simulink library "halin"  (R2021b)
settings: Solver=VariableStepAuto  StartTime=0.0  StopTime=10.0  RelTol=1e-3
undefined symbols (not defined in the file): TRUE
libraries: FVT_lib x37, hcu_lib x31
(part 1 of 4)
settings Model: Creator=13168  LastModifiedBy=FVT23010
settings SolverCC: AlgebraicLoopSolver=TrustRegion
settings DataIOCC: SaveFormat=Array  SignalLoggingSaveFormat=ModelDataLogs  ReturnWorkspaceOutputs=off
settings OptimizationCC: BlockReduction=off  BooleanDataType=off
settings DebuggingCC: SaveWithParameterizedLinksMsg=none  UnderspecifiedInitializationDetection=Classic  MergeDetectMultiDrivingBlocksExec=none  SignalResolutionControl=TryResolveAllWithWarning  SFMachineParentedDataDiag=warning
settings HardwareCC: TargetUnknown=on
settings ModelReferenceCC: PropagateSignalLabelsOutOfModel=off
settings ConfigComp: CovMetricSettings=dw  CovSaveCumulativeToWorkspaceVar=on  CovSaveSingleToWorkspaceVar=on

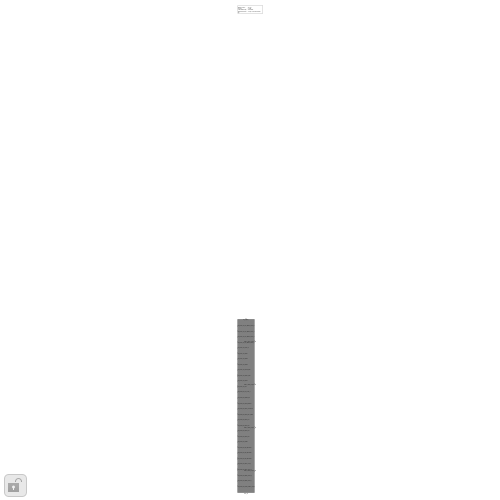
[thumbnail: Simulink's stored preview of the top-level diagram]
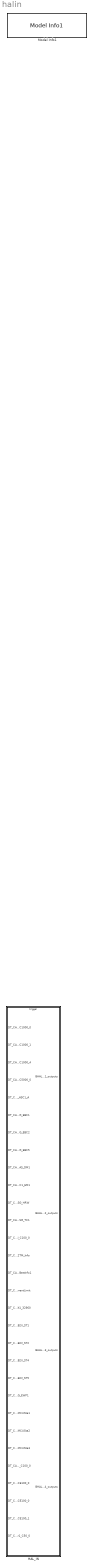
== system halin ==
  HAL_IN : Subsystem
      settings: RTWSystemCode=Nonreusable function  RTWFcnNameOpts=Use subsystem name  RTWFileNameOpts=Use subsystem name
  Model Info1 : hcu_lib/Model Info1  BlockCM=None  Frame=on  DisplayStringWithTags=|  HorizontalTextAlignment=Left  LeftAlignmentValue=0.02  SourceBlockDiagram=hcu_lib  TagMaxNumber=20
      | Model Version        : %<ModelVersion>
      | Creator                   : %<Creator>
      | Last Modified By    : %<LastModifiedBy>
      | Modification date    : %<LastModificationDate>
      settings: SourceProductName=HCU Relative Block Library

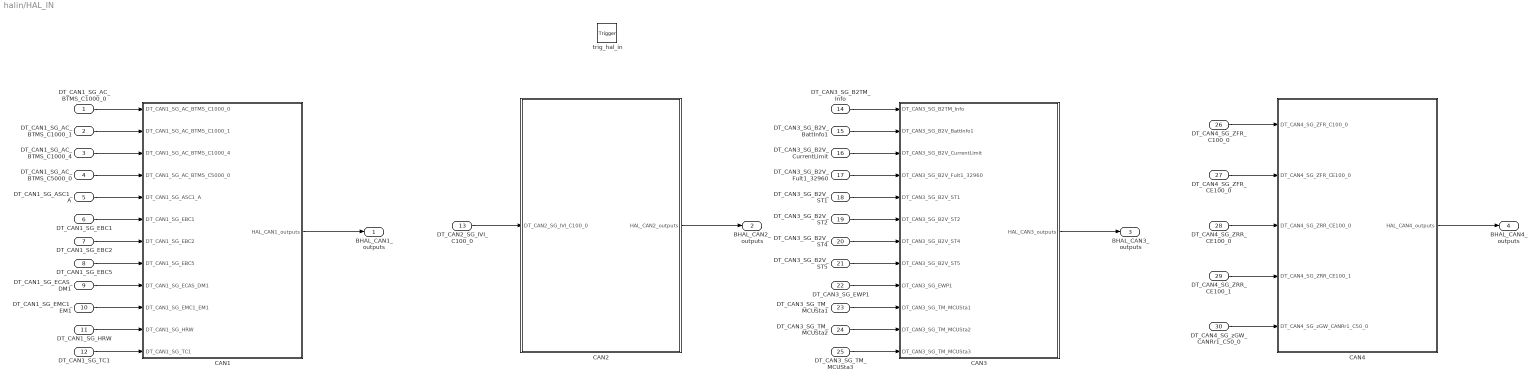
== system halin/HAL_IN ==
  DT_CAN1_SG_AC_BTMS_C1000_0 : Inport
  DT_CAN1_SG_AC_BTMS_C1000_1 : Inport  Port=2
  DT_CAN1_SG_AC_BTMS_C1000_4 : Inport  Port=3
  DT_CAN1_SG_AC_BTMS_C5000_0 : Inport  Port=4
  DT_CAN1_SG_ASC1_A : Inport  Port=5
  DT_CAN1_SG_EBC1 : Inport  Port=6
  DT_CAN1_SG_EBC2 : Inport  Port=7
  DT_CAN1_SG_EBC5 : Inport  Port=8
  DT_CAN1_SG_ECAS_DM1 : Inport  Port=9
  DT_CAN1_SG_EMC1_EM1 : Inport  Port=10
  DT_CAN1_SG_HRW : Inport  Port=11
  DT_CAN1_SG_TC1 : Inport  Port=12
  DT_CAN2_SG_IVI_C100_0 : Inport  Port=13
  DT_CAN3_SG_B2TM_Info : Inport  Port=14
  DT_CAN3_SG_B2V_BattInfo1 : Inport  Port=15
  DT_CAN3_SG_B2V_CurrentLimit : Inport  Port=16
  DT_CAN3_SG_B2V_Fult1_32960 : Inport  Port=17
  DT_CAN3_SG_B2V_ST1 : Inport  Port=18
  DT_CAN3_SG_B2V_ST2 : Inport  Port=19
  DT_CAN3_SG_B2V_ST4 : Inport  Port=20
  DT_CAN3_SG_B2V_ST5 : Inport  Port=21
  DT_CAN3_SG_EWP1 : Inport  Port=22
  DT_CAN3_SG_TM_MCUSta1 : Inport  Port=23
  DT_CAN3_SG_TM_MCUSta2 : Inport  Port=24
  DT_CAN3_SG_TM_MCUSta3 : Inport  Port=25
  DT_CAN4_SG_ZFR_C100_0 : Inport  Port=26
  DT_CAN4_SG_ZFR_CE100_0 : Inport  Port=27
  DT_CAN4_SG_ZRR_CE100_0 : Inport  Port=28
  DT_CAN4_SG_ZRR_CE100_1 : Inport  Port=29
  DT_CAN4_SG_zGW_CANRr1_C50_0 : Inport  Port=30
  trig_hal_in : TriggerPort  TriggerType=function-call  VariantControl=(inherit)
  CAN1 : Subsystem
  CAN2 : Subsystem
  CAN3 : Subsystem
  CAN4 : Subsystem
  BHAL_CAN1_outputs : Outport  OutDataTypeStr=Bus: BHAL_CAN1_outputs
  BHAL_CAN2_outputs : Outport  Port=2  OutDataTypeStr=Bus: BHAL_CAN2_outputs
  BHAL_CAN3_outputs : Outport  Port=3  OutDataTypeStr=Bus: BHAL_CAN3_outputs
  BHAL_CAN4_outputs : Outport  Port=4  OutDataTypeStr=Bus: BHAL_CAN4_outputs
  wires:
  DT_CAN3_SG_TM_MCUSta2/1 -> CAN3/11(DT_CAN3_SG_TM_MCUSta2)
  DT_CAN1_SG_AC_BTMS_C1000_4/1 -> CAN1/3(DT_CAN1_SG_AC_BTMS_C1000_4)
  DT_CAN1_SG_AC_BTMS_C1000_1/1 -> CAN1/2(DT_CAN1_SG_AC_BTMS_C1000_1)
  DT_CAN1_SG_AC_BTMS_C1000_0/1 -> CAN1/1(DT_CAN1_SG_AC_BTMS_C1000_0)
  DT_CAN1_SG_EBC1/1 -> CAN1/6(DT_CAN1_SG_EBC1)
  DT_CAN1_SG_EBC2/1 -> CAN1/7(DT_CAN1_SG_EBC2)
  DT_CAN3_SG_TM_MCUSta3/1 -> CAN3/12(DT_CAN3_SG_TM_MCUSta3)
  DT_CAN1_SG_ASC1_A/1 -> CAN1/5(DT_CAN1_SG_ASC1_A)
  DT_CAN1_SG_HRW/1 -> CAN1/11(DT_CAN1_SG_HRW)
  DT_CAN1_SG_AC_BTMS_C5000_0/1 -> CAN1/4(DT_CAN1_SG_AC_BTMS_C5000_0)
  DT_CAN1_SG_TC1/1 -> CAN1/12(DT_CAN1_SG_TC1)
  DT_CAN1_SG_EMC1_EM1/1 -> CAN1/10(DT_CAN1_SG_EMC1_EM1)
  DT_CAN1_SG_ECAS_DM1/1 -> CAN1/9(DT_CAN1_SG_ECAS_DM1)
  DT_CAN1_SG_EBC5/1 -> CAN1/8(DT_CAN1_SG_EBC5)
  CAN1/1(HAL_CAN1_outputs) -> BHAL_CAN1_outputs/1
  DT_CAN3_SG_B2TM_Info/1 -> CAN3/1(DT_CAN3_SG_B2TM_Info)
  CAN3/1(HAL_CAN3_outputs) -> BHAL_CAN3_outputs/1
  DT_CAN3_SG_B2V_ST5/1 -> CAN3/8(DT_CAN3_SG_B2V_ST5)
  DT_CAN3_SG_B2V_ST4/1 -> CAN3/7(DT_CAN3_SG_B2V_ST4)
  DT_CAN3_SG_B2V_CurrentLimit/1 -> CAN3/3(DT_CAN3_SG_B2V_CurrentLimit)
  DT_CAN3_SG_EWP1/1 -> CAN3/9(DT_CAN3_SG_EWP1)
  CAN2/1(HAL_CAN2_outputs) -> BHAL_CAN2_outputs/1
  DT_CAN3_SG_B2V_ST2/1 -> CAN3/6(DT_CAN3_SG_B2V_ST2)
  DT_CAN3_SG_B2V_ST1/1 -> CAN3/5(DT_CAN3_SG_B2V_ST1)
  DT_CAN4_SG_ZFR_C100_0/1 -> CAN4/1(DT_CAN4_SG_ZFR_C100_0)
  CAN4/1(HAL_CAN4_outputs) -> BHAL_CAN4_outputs/1
  DT_CAN4_SG_ZFR_CE100_0/1 -> CAN4/2(DT_CAN4_SG_ZFR_CE100_0)
  DT_CAN3_SG_TM_MCUSta1/1 -> CAN3/10(DT_CAN3_SG_TM_MCUSta1)
  DT_CAN2_SG_IVI_C100_0/1 -> CAN2/1(DT_CAN2_SG_IVI_C100_0)
  DT_CAN4_SG_zGW_CANRr1_C50_0/1 -> CAN4/5(DT_CAN4_SG_zGW_CANRr1_C50_0)
  DT_CAN4_SG_ZRR_CE100_1/1 -> CAN4/4(DT_CAN4_SG_ZRR_CE100_1)
  DT_CAN4_SG_ZRR_CE100_0/1 -> CAN4/3(DT_CAN4_SG_ZRR_CE100_0)
  DT_CAN3_SG_B2V_Fult1_32960/1 -> CAN3/4(DT_CAN3_SG_B2V_Fult1_32960)
  DT_CAN3_SG_B2V_BattInfo1/1 -> CAN3/2(DT_CAN3_SG_B2V_BattInfo1)

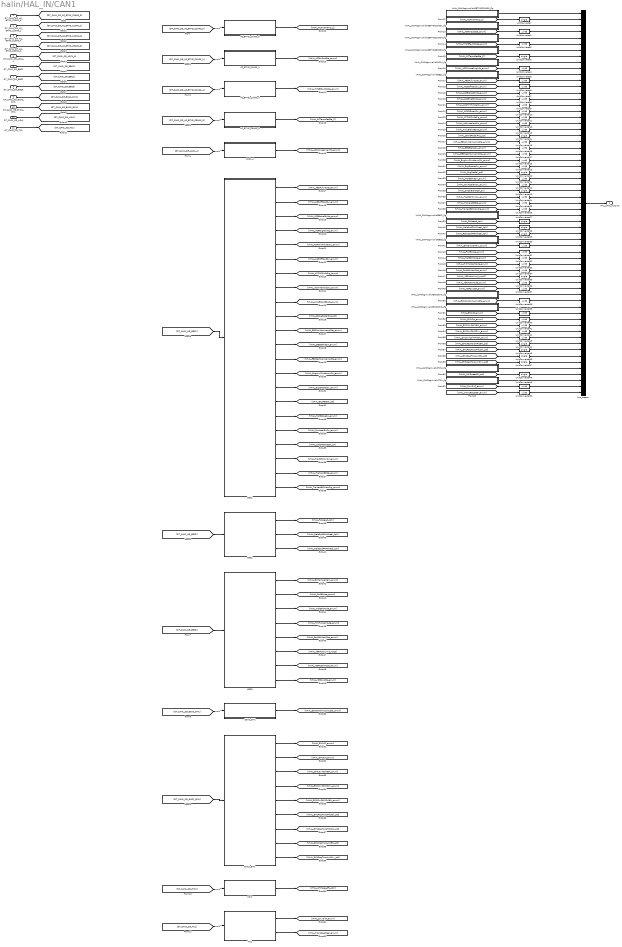
== system halin/HAL_IN/CAN1 ==
  DT_CAN1_SG_AC_BTMS_C1000_0 : Inport
  DT_CAN1_SG_AC_BTMS_C1000_1 : Inport  Port=2
  DT_CAN1_SG_AC_BTMS_C1000_4 : Inport  Port=3
  DT_CAN1_SG_AC_BTMS_C5000_0 : Inport  Port=4
  DT_CAN1_SG_ASC1_A : Inport  Port=5
  DT_CAN1_SG_EBC1 : Inport  Port=6
  DT_CAN1_SG_EBC2 : Inport  Port=7
  DT_CAN1_SG_EBC5 : Inport  Port=8
  DT_CAN1_SG_ECAS_DM1 : Inport  Port=9
  DT_CAN1_SG_EMC1_EM1 : Inport  Port=10
  DT_CAN1_SG_HRW : Inport  Port=11
  DT_CAN1_SG_TC1 : Inport  Port=12
  AC_BTMS_C1000_0 : Subsystem
  AC_BTMS_C1000_1 : Subsystem
  AC_BTMS_C1000_4 : Subsystem
  AC_BTMS_C5000_0 : Subsystem
  ASC1_A : Subsystem
  EBC1 : Subsystem
  EBC2 : Subsystem
  EBC5 : Subsystem
  ECAS_DM1 : Subsystem
  EMC1_EM1 : Subsystem
  HRW : Subsystem
  TC1 : Subsystem
  UnitConverter{,3,14,20,23,27..29,35,44..48} (14 alike) : DataTypeConversion  OutDataTypeStr=single
  UnitConverter{1..2,4..13,15..19,21..22,24..26,30..34,36..43,49..50} (37 alike) : DataTypeConversion  OutDataTypeStr=uint8
  VHAL_CANMsgInvalidACBTMSC10000_flg : Subsystem  AncestorBlock=FVT_lib/hal/MsgTimeoutJudge_CAN_AUTOSAR
      mask help: MeasumentTrigerEvent
      mask Display: fprintf('MsgTimeoutJudge_CAN\nAUTOSAR');
  VHAL_CANMsgInvalidACBTMSC10001_flg : Subsystem  AncestorBlock=FVT_lib/hal/MsgTimeoutJudge_CAN_AUTOSAR
      mask help: MeasumentTrigerEvent
      mask Display: fprintf('MsgTimeoutJudge_CAN\nAUTOSAR');
  VHAL_CANMsgInvalidACBTMSC10004_flg : Subsystem  AncestorBlock=FVT_lib/hal/MsgTimeoutJudge_CAN_AUTOSAR
      mask help: MeasumentTrigerEvent
      mask Display: fprintf('MsgTimeoutJudge_CAN\nAUTOSAR');
  VHAL_CANMsgInvalidACBTMSC50000_flg : Subsystem  AncestorBlock=FVT_lib/hal/MsgTimeoutJudge_CAN_AUTOSAR
      mask help: MeasumentTrigerEvent
      mask Display: fprintf('MsgTimeoutJudge_CAN\nAUTOSAR');
  VHAL_CANMsgInvalidASC1A_flg : Subsystem  AncestorBlock=FVT_lib/hal/MsgTimeoutJudge_CAN_AUTOSAR
      mask help: MeasumentTrigerEvent
      mask Display: fprintf('MsgTimeoutJudge_CAN\nAUTOSAR');
  VHAL_CANMsgInvalidEBC1_flg : Subsystem  AncestorBlock=FVT_lib/hal/MsgTimeoutJudge_CAN_AUTOSAR
      mask help: MeasumentTrigerEvent
      mask Display: fprintf('MsgTimeoutJudge_CAN\nAUTOSAR');
  VHAL_CANMsgInvalidEBC2_flg : Subsystem  AncestorBlock=FVT_lib/hal/MsgTimeoutJudge_CAN_AUTOSAR
      mask help: MeasumentTrigerEvent
      mask Display: fprintf('MsgTimeoutJudge_CAN\nAUTOSAR');
  VHAL_CANMsgInvalidEBC5_flg : Subsystem  AncestorBlock=FVT_lib/hal/MsgTimeoutJudge_CAN_AUTOSAR
      mask help: MeasumentTrigerEvent
      mask Display: fprintf('MsgTimeoutJudge_CAN\nAUTOSAR');
  VHAL_CANMsgInvalidECASDM1_flg : Subsystem  AncestorBlock=FVT_lib/hal/MsgTimeoutJudge_CAN_AUTOSAR
      mask help: MeasumentTrigerEvent
      mask Display: fprintf('MsgTimeoutJudge_CAN\nAUTOSAR');
  VHAL_CANMsgInvalidEMC1EM1_flg : Subsystem  AncestorBlock=FVT_lib/hal/MsgTimeoutJudge_CAN_AUTOSAR
      mask help: MeasumentTrigerEvent
      mask Display: fprintf('MsgTimeoutJudge_CAN\nAUTOSAR');
  VHAL_CANMsgInvalidHRW_flg : Subsystem  AncestorBlock=FVT_lib/hal/MsgTimeoutJudge_CAN_AUTOSAR
      mask help: MeasumentTrigerEvent
      mask Display: fprintf('MsgTimeoutJudge_CAN\nAUTOSAR');
  VHAL_CANMsgInvalidTC1_flg : Subsystem  AncestorBlock=FVT_lib/hal/MsgTimeoutJudge_CAN_AUTOSAR
      mask help: MeasumentTrigerEvent
      mask Display: fprintf('MsgTimeoutJudge_CAN\nAUTOSAR');
  bus_creator : BusCreator  Inputs=63  OutDataTypeStr=Bus: BHAL_CAN1_outputs  NonVirtualBus=on
  HAL_CAN1_outputs : Outport
  wires:
  DT_CAN1_SG_AC_BTMS_C1000_0/1 -> [DT_CAN1_SG_AC_BTMS_C1000_0]
  DT_CAN1_SG_AC_BTMS_C1000_1/1 -> [DT_CAN1_SG_AC_BTMS_C1000_1]
  DT_CAN1_SG_AC_BTMS_C1000_4/1 -> [DT_CAN1_SG_AC_BTMS_C1000_4]
  DT_CAN1_SG_AC_BTMS_C5000_0/1 -> [DT_CAN1_SG_AC_BTMS_C5000_0]
  DT_CAN1_SG_ASC1_A/1 -> [DT_CAN1_SG_ASC1_A]
  DT_CAN1_SG_EBC1/1 -> [DT_CAN1_SG_EBC1]
  DT_CAN1_SG_EBC2/1 -> [DT_CAN1_SG_EBC2]
  DT_CAN1_SG_EBC5/1 -> [DT_CAN1_SG_EBC5]
  DT_CAN1_SG_ECAS_DM1/1 -> [DT_CAN1_SG_ECAS_DM1]
  DT_CAN1_SG_EMC1_EM1/1 -> [DT_CAN1_SG_EMC1_EM1]
  DT_CAN1_SG_HRW/1 -> [DT_CAN1_SG_HRW]
  DT_CAN1_SG_TC1/1 -> [DT_CAN1_SG_TC1]
  [DT_CAN1_SG_AC_BTMS_C1000_0] -> AC_BTMS_C1000_0/1(DT_CAN1_SG_AC_BTMS_C1000_0)
  [DT_CAN1_SG_AC_BTMS_C1000_1] -> AC_BTMS_C1000_1/1(DT_CAN1_SG_AC_BTMS_C1000_1)
  [DT_CAN1_SG_AC_BTMS_C1000_4] -> AC_BTMS_C1000_4/1(DT_CAN1_SG_AC_BTMS_C1000_4)
  [DT_CAN1_SG_AC_BTMS_C5000_0] -> AC_BTMS_C5000_0/1(DT_CAN1_SG_AC_BTMS_C5000_0)
  [DT_CAN1_SG_ASC1_A] -> ASC1_A/1(DT_CAN1_SG_ASC1_A)
  [DT_CAN1_SG_EBC1] -> EBC1/1(DT_CAN1_SG_EBC1)
  [DT_CAN1_SG_EBC2] -> EBC2/1(DT_CAN1_SG_EBC2)
  [DT_CAN1_SG_EBC5] -> EBC5/1(DT_CAN1_SG_EBC5)
  [DT_CAN1_SG_ECAS_DM1] -> ECAS_DM1/1(DT_CAN1_SG_ECAS_DM1)
  [DT_CAN1_SG_EMC1_EM1] -> EMC1_EM1/1(DT_CAN1_SG_EMC1_EM1)
  [DT_CAN1_SG_HRW] -> HRW/1(DT_CAN1_SG_HRW)
  [DT_CAN1_SG_TC1] -> TC1/1(DT_CAN1_SG_TC1)
  bus_creator/1 -> HAL_CAN1_outputs/1
  VHAL_CANMsgInvalidACBTMSC10000_flg/1(Out) -> bus_creator/1
  AC_BTMS_C1000_0/1(VHAL_ACAmbTemp_C) -> [VHAL_ACAmbTemp_C]
  UnitConverter/1 -> bus_creator/2  "VHAL_ACAmbTemp_C"
  [VHAL_ACAmbTemp_C] -> UnitConverter/1
  VHAL_CANMsgInvalidACBTMSC10001_flg/1(Out) -> bus_creator/3
  AC_BTMS_C1000_1/1(VHAL_ACFanSpdSta_enum) -> [VHAL_ACFanSpdSta_enum]
  UnitConverter1/1 -> bus_creator/4  "VHAL_ACFanSpdSta_enum"
  [VHAL_ACFanSpdSta_enum] -> UnitConverter1/1
  VHAL_CANMsgInvalidACBTMSC10004_flg/1(Out) -> bus_creator/5
  AC_BTMS_C1000_4/1(VHAL_TM2BFaultCode_enum) -> [VHAL_TM2BFaultCode_enum]
  UnitConverter2/1 -> bus_creator/6  "VHAL_TM2BFaultCode_enum"
  [VHAL_TM2BFaultCode_enum] -> UnitConverter2/1
  VHAL_CANMsgInvalidACBTMSC50000_flg/1(Out) -> bus_creator/7
  AC_BTMS_C5000_0/1(VHAL_ACTempSetSta_C) -> [VHAL_ACTempSetSta_C]
  UnitConverter3/1 -> bus_creator/8  "VHAL_ACTempSetSta_C"
  [VHAL_ACTempSetSta_C] -> UnitConverter3/1
  VHAL_CANMsgInvalidASC1A_flg/1(Out) -> bus_creator/9
  ASC1_A/1(VHAL_ASC1KneelingInfo_enum) -> [VHAL_ASC1KneelingInfo_enum]
  UnitConverter4/1 -> bus_creator/10  "VHAL_ASC1KneelingInfo_enum"
  [VHAL_ASC1KneelingInfo_enum] -> UnitConverter4/1
  VHAL_CANMsgInvalidEBC1_flg/1(Out) -> bus_creator/11
  EBC1/1(VHAL_ABSFullyOper_enum) -> [VHAL_ABSFullyOper_enum]
  UnitConverter5/1 -> bus_creator/12  "VHAL_ABSFullyOper_enum"
  [VHAL_ABSFullyOper_enum] -> UnitConverter5/1
  EBC1/2(VHAL_ABSOffroadSw_enum) -> [VHAL_ABSOffroadSw_enum]
  UnitConverter6/1 -> bus_creator/13  "VHAL_ABSOffroadSw_enum"
  [VHAL_ABSOffroadSw_enum] -> UnitConverter6/1
  EBC1/3(VHAL_ASRBrakeCtrlAtc_enum) -> [VHAL_ASRBrakeCtrlAtc_enum]
  UnitConverter7/1 -> bus_creator/14  "VHAL_ASRBrakeCtrlAtc_enum"
  [VHAL_ASRBrakeCtrlAtc_enum] -> UnitConverter7/1
  EBC1/4(VHAL_ASREngCtrlAtc_enum) -> [VHAL_ASREngCtrlAtc_enum]
  UnitConverter8/1 -> bus_creator/15  "VHAL_ASREngCtrlAtc_enum"
  [VHAL_ASREngCtrlAtc_enum] -> UnitConverter8/1
  EBC1/5(VHAL_ASRHillHolderSw_enum) -> [VHAL_ASRHillHolderSw_enum]
  UnitConverter9/1 -> bus_creator/16  "VHAL_ASRHillHolderSw_enum"
  [VHAL_ASRHillHolderSw_enum] -> UnitConverter9/1
  EBC1/6(VHAL_ASROffroadSw_enum) -> [VHAL_ASROffroadSw_enum]
  UnitConverter10/1 -> bus_creator/17  "VHAL_ASROffroadSw_enum"
  [VHAL_ASROffroadSw_enum] -> UnitConverter10/1
  EBC1/7(VHAL_ATCASRInfoSig_enum) -> [VHAL_ATCASRInfoSig_enum]
  UnitConverter11/1 -> bus_creator/18  "VHAL_ATCASRInfoSig_enum"
  [VHAL_ATCASRInfoSig_enum] -> UnitConverter11/1
  EBC1/8(VHAL_AcltrInterlockSw_enum) -> [VHAL_AcltrInterlockSw_enum]
  UnitConverter12/1 -> bus_creator/19  "VHAL_AcltrInterlockSw_enum"
  [VHAL_AcltrInterlockSw_enum] -> UnitConverter12/1
  EBC1/9(VHAL_AntiLBrakABSAct_enum) -> [VHAL_AntiLBrakABSAct_enum]
  UnitConverter13/1 -> bus_creator/20  "VHAL_AntiLBrakABSAct_enum"
  [VHAL_AntiLBrakABSAct_enum] -> UnitConverter13/1
  EBC1/10(VHAL_BrakePedalPos_pct) -> [VHAL_BrakePedalPos_pct]
  UnitConverter14/1 -> bus_creator/21  "VHAL_BrakePedalPos_pct"
  [VHAL_BrakePedalPos_pct] -> UnitConverter14/1
  EBC1/11(VHAL_EBSAmWarnLampSta_enum) -> [VHAL_EBSAmWarnLampSta_enum]
  UnitConverter15/1 -> bus_creator/22  "VHAL_EBSAmWarnLampSta_enum"
  [VHAL_EBSAmWarnLampSta_enum] -> UnitConverter15/1
  EBC1/12(VHAL_EBSBrakeSw_enum) -> [VHAL_EBSBrakeSw_enum]
  UnitConverter16/1 -> bus_creator/23  "VHAL_EBSBrakeSw_enum"
  [VHAL_EBSBrakeSw_enum] -> UnitConverter16/1
  EBC1/13(VHAL_EBSRedWarnLampSta_enum) -> [VHAL_EBSRedWarnLampSta_enum]
  UnitConverter17/1 -> bus_creator/24  "VHAL_EBSRedWarnLampSta_enum"
  [VHAL_EBSRedWarnLampSta_enum] -> UnitConverter17/1
  EBC1/14(VHAL_EngAuxShutdownSw_enum) -> [VHAL_EngAuxShutdownSw_enum]
  UnitConverter18/1 -> bus_creator/25  "VHAL_EngAuxShutdownSw_enum"
  [VHAL_EngAuxShutdownSw_enum] -> UnitConverter18/1
  EBC1/15(VHAL_EngDerateSw_enum) -> [VHAL_EngDerateSw_enum]
  UnitConverter19/1 -> bus_creator/26  "VHAL_EngDerateSw_enum"
  [VHAL_EngDerateSw_enum] -> UnitConverter19/1
  EBC1/16(VHAL_EngRetSel_pct) -> [VHAL_EngRetSel_pct]
  UnitConverter20/1 -> bus_creator/27  "VHAL_EngRetSel_pct"
  [VHAL_EngRetSel_pct] -> UnitConverter20/1
  EBC1/17(VHAL_HaltBrakeSw_enum) -> [VHAL_HaltBrakeSw_enum]
  UnitConverter21/1 -> bus_creator/28  "VHAL_HaltBrakeSw_enum"
  [VHAL_HaltBrakeSw_enum] -> UnitConverter21/1
  EBC1/18(VHAL_RmAccelEnSw_enum) -> [VHAL_RmAccelEnSw_enum]
  UnitConverter22/1 -> bus_creator/29  "VHAL_RmAccelEnSw_enum"
  [VHAL_RmAccelEnSw_enum] -> UnitConverter22/1
  EBC1/19(VHAL_SACtrlBrakeCtrl_SA) -> [VHAL_SACtrlBrakeCtrl_SA]
  UnitConverter23/1 -> bus_creator/30  "VHAL_SACtrlBrakeCtrl_SA"
  [VHAL_SACtrlBrakeCtrl_SA] -> UnitConverter23/1
  EBC1/20(VHAL_TractCtrlOvrSw_enum) -> [VHAL_TractCtrlOvrSw_enum]
  UnitConverter24/1 -> bus_creator/31  "VHAL_TractCtrlOvrSw_enum"
  [VHAL_TractCtrlOvrSw_enum] -> UnitConverter24/1
  EBC1/21(VHAL_TrailerABSSta_enum) -> [VHAL_TrailerABSSta_enum]
  UnitConverter25/1 -> bus_creator/32  "VHAL_TrailerABSSta_enum"
  [VHAL_TrailerABSSta_enum] -> UnitConverter25/1
  EBC1/22(VHAL_TrailerABSWarnSig_enum) -> [VHAL_TrailerABSWarnSig_enum]
  UnitConverter26/1 -> bus_creator/33  "VHAL_TrailerABSWarnSig_enum"
  [VHAL_TrailerABSWarnSig_enum] -> UnitConverter26/1
  VHAL_CANMsgInvalidEBC2_flg/1(Out) -> bus_creator/34
  EBC2/1(VHAL_FASpeed_kph) -> [VHAL_FASpeed_kph]
  UnitConverter27/1 -> bus_creator/35  "VHAL_FASpeed_kph"
  [VHAL_FASpeed_kph] -> UnitConverter27/1
  EBC2/2(VHAL_RelaSpdFALWheel_kph) -> [VHAL_RelaSpdFALWheel_kph]
  UnitConverter28/1 -> bus_creator/36  "VHAL_RelaSpdFALWheel_kph"
  [VHAL_RelaSpdFALWheel_kph] -> UnitConverter28/1
  EBC2/3(VHAL_RelaSpdFARWheel_kph) -> [VHAL_RelaSpdFARWheel_kph]
  UnitConverter29/1 -> bus_creator/37  "VHAL_RelaSpdFARWheel_kph"
  [VHAL_RelaSpdFARWheel_kph] -> UnitConverter29/1
  VHAL_CANMsgInvalidEBC5_flg/1(Out) -> bus_creator/38
  EBC5/1(VHAL_BrkTempeWarn_enum) -> [VHAL_BrkTempeWarn_enum]
  UnitConverter30/1 -> bus_creator/39  "VHAL_BrkTempeWarn_enum"
  [VHAL_BrkTempeWarn_enum] -> UnitConverter30/1
  EBC5/2(VHAL_FndBrkUse_enum) -> [VHAL_FndBrkUse_enum]
  UnitConverter31/1 -> bus_creator/40  "VHAL_FndBrkUse_enum"
  [VHAL_FndBrkUse_enum] -> UnitConverter31/1
  EBC5/3(VHAL_HaltBrkMode_enum) -> [VHAL_HaltBrkMode_enum]
  UnitConverter32/1 -> bus_creator/41  "VHAL_HaltBrkMode_enum"
  [VHAL_HaltBrkMode_enum] -> UnitConverter32/1
  EBC5/4(VHAL_HillHolderMode_enum) -> [VHAL_HillHolderMode_enum]
  UnitConverter33/1 -> bus_creator/42  "VHAL_HillHolderMode_enum"
  [VHAL_HillHolderMode_enum] -> UnitConverter33/1
  EBC5/5(VHAL_ParkBrkActuFAct_enum) -> [VHAL_ParkBrkActuFAct_enum]
  UnitConverter34/1 -> bus_creator/43  "VHAL_ParkBrkActuFAct_enum"
  [VHAL_ParkBrkActuFAct_enum] -> UnitConverter34/1
  EBC5/6(VHAL_XBRAcltnLimit_mps2) -> [VHAL_XBRAcltnLimit_mps2]
  UnitConverter35/1 -> bus_creator/44  "VHAL_XBRAcltnLimit_mps2"
  [VHAL_XBRAcltnLimit_mps2] -> UnitConverter35/1
  EBC5/7(VHAL_XBRActtrlMode_enum) -> [VHAL_XBRActtrlMode_enum]
  UnitConverter36/1 -> bus_creator/45  "VHAL_XBRActtrlMode_enum"
  [VHAL_XBRActtrlMode_enum] -> UnitConverter36/1
  EBC5/8(VHAL_XBRSysSta_enum) -> [VHAL_XBRSysSta_enum]
  UnitConverter37/1 -> bus_creator/46  "VHAL_XBRSysSta_enum"
  [VHAL_XBRSysSta_enum] -> UnitConverter37/1
  VHAL_CANMsgInvalidECASDM1_flg/1(Out) -> bus_creator/47
  ECAS_DM1/1(VHAL_ECASAWarmLampSta_enum) -> [VHAL_ECASAWarmLampSta_enum]
  UnitConverter38/1 -> bus_creator/48  "VHAL_ECASAWarmLampSta_enum"
  [VHAL_ECASAWarmLampSta_enum] -> UnitConverter38/1
  VHAL_CANMsgInvalidEMC1EM1_flg/1(Out) -> bus_creator/49
  EMC1_EM1/1(VHAL_EM1CS_enum) -> [VHAL_EM1CS_enum]
  UnitConverter39/1 -> bus_creator/50  "VHAL_EM1CS_enum"
  [VHAL_EM1CS_enum] -> UnitConverter39/1
  EMC1_EM1/2(VHAL_EM1Cnt_enum) -> [VHAL_EM1Cnt_enum]
  UnitConverter40/1 -> bus_creator/51  "VHAL_EM1Cnt_enum"
  [VHAL_EM1Cnt_enum] -> UnitConverter40/1
  EMC1_EM1/3(VHAL_EM1OvrCtrlMBrk_enum) -> [VHAL_EM1OvrCtrlMBrk_enum]
  UnitConverter41/1 -> bus_creator/52  "VHAL_EM1OvrCtrlMBrk_enum"
  [VHAL_EM1OvrCtrlMBrk_enum] -> UnitConverter41/1
  EMC1_EM1/4(VHAL_EM1OvrCtrlMDriv_enum) -> [VHAL_EM1OvrCtrlMDriv_enum]
  UnitConverter42/1 -> bus_creator/53  "VHAL_EM1OvrCtrlMDriv_enum"
  [VHAL_EM1OvrCtrlMDriv_enum] -> UnitConverter42/1
  EMC1_EM1/5(VHAL_EM1OvrCtrlMPriBrk_enum) -> [VHAL_EM1OvrCtrlMPriBrk_enum]
  UnitConverter43/1 -> bus_creator/54  "VHAL_EM1OvrCtrlMPriBrk_enum"
  [VHAL_EM1OvrCtrlMPriBrk_enum] -> UnitConverter43/1
  EMC1_EM1/6(VHAL_EM1ReqTorqHRlsBrk_pct) -> [VHAL_EM1ReqTorqHRlsBrk_pct]
  UnitConverter44/1 -> bus_creator/55  "VHAL_EM1ReqTorqHRlsBrk_pct"
  [VHAL_EM1ReqTorqHRlsBrk_pct] -> UnitConverter44/1
  EMC1_EM1/7(VHAL_EM1ReqTorqHRlsDri_pct) -> [VHAL_EM1ReqTorqHRlsDri_pct]
  UnitConverter45/1 -> bus_creator/56  "VHAL_EM1ReqTorqHRlsDri_pct"
  [VHAL_EM1ReqTorqHRlsDri_pct] -> UnitConverter45/1
  EMC1_EM1/8(VHAL_EM1ReqTorqLimBrk_pct) -> [VHAL_EM1ReqTorqLimBrk_pct]
  UnitConverter46/1 -> bus_creator/57  "VHAL_EM1ReqTorqLimBrk_pct"
  [VHAL_EM1ReqTorqLimBrk_pct] -> UnitConverter46/1
  EMC1_EM1/9(VHAL_EM1ReqTorqLimDriv_pct) -> [VHAL_EM1ReqTorqLimDriv_pct]
  UnitConverter47/1 -> bus_creator/58  "VHAL_EM1ReqTorqLimDriv_pct"
  [VHAL_EM1ReqTorqLimDriv_pct] -> UnitConverter47/1
  VHAL_CANMsgInvalidHRW_flg/1(Out) -> bus_creator/59
  HRW/1(VHAL_WhlSpeedFL_kph) -> [VHAL_WhlSpeedFL_kph]
  UnitConverter48/1 -> bus_creator/60  "VHAL_WhlSpeedFL_kph"
  [VHAL_WhlSpeedFL_kph] -> UnitConverter48/1
  VHAL_CANMsgInvalidTC1_flg/1(Out) -> bus_creator/61
  TC1/1(VHAL_DrivDirF_enum) -> [VHAL_DrivDirF_enum]
  UnitConverter49/1 -> bus_creator/62  "VHAL_DrivDirF_enum"
  [VHAL_DrivDirF_enum] -> UnitConverter49/1
  TC1/2(VHAL_TransReqGear_enum) -> [VHAL_TransReqGear_enum]
  UnitConverter50/1 -> bus_creator/63  "VHAL_TransReqGear_enum"
  [VHAL_TransReqGear_enum] -> UnitConverter50/1

== system halin/HAL_IN/CAN2 ==
  DT_CAN2_SG_IVI_C100_0 : Inport
  IVI_C100_0 : Subsystem
  UnitConverter : DataTypeConversion  OutDataTypeStr=uint8
  VHAL_CANMsgInvalidIVIC1000_flg : Subsystem  AncestorBlock=FVT_lib/hal/MsgTimeoutJudge_CAN_AUTOSAR
      mask help: MeasumentTrigerEvent
      mask Display: fprintf('MsgTimeoutJudge_CAN\nAUTOSAR');
  bus_creator : BusCreator  Inputs=2  OutDataTypeStr=Bus: BHAL_CAN2_outputs  NonVirtualBus=on
  HAL_CAN2_outputs : Outport
  wires:
  DT_CAN2_SG_IVI_C100_0/1 -> [DT_CAN2_SG_IVI_C100_0]
  [DT_CAN2_SG_IVI_C100_0] -> IVI_C100_0/1(DT_CAN2_SG_IVI_C100_0)
  bus_creator/1 -> HAL_CAN2_outputs/1
  VHAL_CANMsgInvalidIVIC1000_flg/1(Out) -> bus_creator/1
  IVI_C100_0/1(VHAL_IVIACFanSpdReqCmd_enum) -> [VHAL_IVIACFanSpdReqCmd_enum]
  UnitConverter/1 -> bus_creator/2  "VHAL_IVIACFanSpdReqCmd_enum"
  [VHAL_IVIACFanSpdReqCmd_enum] -> UnitConverter/1

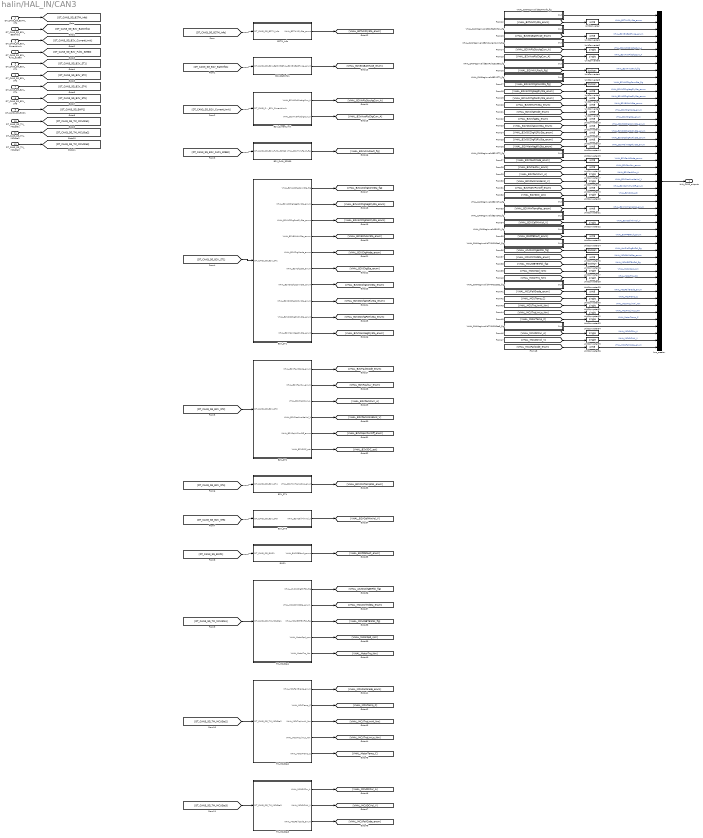
== system halin/HAL_IN/CAN3 ==
  DT_CAN3_SG_B2TM_Info : Inport
  DT_CAN3_SG_B2V_BattInfo1 : Inport  Port=2
  DT_CAN3_SG_B2V_CurrentLimit : Inport  Port=3
  DT_CAN3_SG_B2V_Fult1_32960 : Inport  Port=4
  DT_CAN3_SG_B2V_ST1 : Inport  Port=5
  DT_CAN3_SG_B2V_ST2 : Inport  Port=6
  DT_CAN3_SG_B2V_ST4 : Inport  Port=7
  DT_CAN3_SG_B2V_ST5 : Inport  Port=8
  DT_CAN3_SG_EWP1 : Inport  Port=9
  DT_CAN3_SG_TM_MCUSta1 : Inport  Port=10
  DT_CAN3_SG_TM_MCUSta2 : Inport  Port=11
  DT_CAN3_SG_TM_MCUSta3 : Inport  Port=12
  B2TM_Info : Subsystem
  B2V_BattInfo1 : Subsystem
  B2V_CurrentLimit : Subsystem
  B2V_Fult1_32960 : Subsystem
  B2V_ST1 : Subsystem
  B2V_ST2 : Subsystem
  B2V_ST4 : Subsystem
  B2V_ST5 : Subsystem
  EWP1 : Subsystem
  TM_MCUSta1 : Subsystem
  TM_MCUSta2 : Subsystem
  TM_MCUSta3 : Subsystem
  UnitConverter{,1,6..16,19,21,23,25,29,36} (19 alike) : DataTypeConversion  OutDataTypeStr=uint8
  UnitConverter{2..3,17..18,20,22,27..28,30..35} (14 alike) : DataTypeConversion  OutDataTypeStr=single
  UnitConverter{4..5,24,26} (4 alike) : DataTypeConversion  OutDataTypeStr=boolean
  VHAL_CANMsgInvalidB2TMInfo_flg : Subsystem  AncestorBlock=FVT_lib/hal/MsgTimeoutJudge_CAN_AUTOSAR
      mask help: MeasumentTrigerEvent
      mask Display: fprintf('MsgTimeoutJudge_CAN\nAUTOSAR');
  VHAL_CANMsgInvalidB2VBattInfo1_flg : Subsystem  AncestorBlock=FVT_lib/hal/MsgTimeoutJudge_CAN_AUTOSAR
      mask help: MeasumentTrigerEvent
      mask Display: fprintf('MsgTimeoutJudge_CAN\nAUTOSAR');
  VHAL_CANMsgInvalidB2VCurrentLimit_flg : Subsystem  AncestorBlock=FVT_lib/hal/MsgTimeoutJudge_CAN_AUTOSAR
      mask help: MeasumentTrigerEvent
      mask Display: fprintf('MsgTimeoutJudge_CAN\nAUTOSAR');
  VHAL_CANMsgInvalidB2VFult132960_flg : Subsystem  AncestorBlock=FVT_lib/hal/MsgTimeoutJudge_CAN_AUTOSAR
      mask help: MeasumentTrigerEvent
      mask Display: fprintf('MsgTimeoutJudge_CAN\nAUTOSAR');
  VHAL_CANMsgInvalidB2VST1_flg : Subsystem  AncestorBlock=FVT_lib/hal/MsgTimeoutJudge_CAN_AUTOSAR
      mask help: MeasumentTrigerEvent
      mask Display: fprintf('MsgTimeoutJudge_CAN\nAUTOSAR');
  VHAL_CANMsgInvalidB2VST2_flg : Subsystem  AncestorBlock=FVT_lib/hal/MsgTimeoutJudge_CAN_AUTOSAR
      mask help: MeasumentTrigerEvent
      mask Display: fprintf('MsgTimeoutJudge_CAN\nAUTOSAR');
  VHAL_CANMsgInvalidB2VST4_flg : Subsystem  AncestorBlock=FVT_lib/hal/MsgTimeoutJudge_CAN_AUTOSAR
      mask help: MeasumentTrigerEvent
      mask Display: fprintf('MsgTimeoutJudge_CAN\nAUTOSAR');
  VHAL_CANMsgInvalidB2VST5_flg : Subsystem  AncestorBlock=FVT_lib/hal/MsgTimeoutJudge_CAN_AUTOSAR
      mask help: MeasumentTrigerEvent
      mask Display: fprintf('MsgTimeoutJudge_CAN\nAUTOSAR');
  VHAL_CANMsgInvalidEWP1_flg : Subsystem  AncestorBlock=FVT_lib/hal/MsgTimeoutJudge_CAN_AUTOSAR
      mask help: MeasumentTrigerEvent
      mask Display: fprintf('MsgTimeoutJudge_CAN\nAUTOSAR');
  VHAL_CANMsgInvalidTMMCUSta1_flg : Subsystem  AncestorBlock=FVT_lib/hal/MsgTimeoutJudge_CAN_AUTOSAR
      mask help: MeasumentTrigerEvent
      mask Display: fprintf('MsgTimeoutJudge_CAN\nAUTOSAR');
  VHAL_CANMsgInvalidTMMCUSta2_flg : Subsystem  AncestorBlock=FVT_lib/hal/MsgTimeoutJudge_CAN_AUTOSAR
      mask help: MeasumentTrigerEvent
      mask Display: fprintf('MsgTimeoutJudge_CAN\nAUTOSAR');
  VHAL_CANMsgInvalidTMMCUSta3_flg : Subsystem  AncestorBlock=FVT_lib/hal/MsgTimeoutJudge_CAN_AUTOSAR
      mask help: MeasumentTrigerEvent
      mask Display: fprintf('MsgTimeoutJudge_CAN\nAUTOSAR');
  bus_creator : BusCreator  Inputs=49  OutDataTypeStr=Bus: BHAL_CAN3_outputs  NonVirtualBus=on
  HAL_CAN3_outputs : Outport
  wires:
  DT_CAN3_SG_B2TM_Info/1 -> [DT_CAN3_SG_B2TM_Info]
  DT_CAN3_SG_B2V_BattInfo1/1 -> [DT_CAN3_SG_B2V_BattInfo1]
  DT_CAN3_SG_B2V_CurrentLimit/1 -> [DT_CAN3_SG_B2V_CurrentLimit]
  DT_CAN3_SG_B2V_Fult1_32960/1 -> [DT_CAN3_SG_B2V_Fult1_32960]
  DT_CAN3_SG_B2V_ST1/1 -> [DT_CAN3_SG_B2V_ST1]
  DT_CAN3_SG_B2V_ST2/1 -> [DT_CAN3_SG_B2V_ST2]
  DT_CAN3_SG_B2V_ST4/1 -> [DT_CAN3_SG_B2V_ST4]
  DT_CAN3_SG_B2V_ST5/1 -> [DT_CAN3_SG_B2V_ST5]
  DT_CAN3_SG_EWP1/1 -> [DT_CAN3_SG_EWP1]
  DT_CAN3_SG_TM_MCUSta1/1 -> [DT_CAN3_SG_TM_MCUSta1]
  DT_CAN3_SG_TM_MCUSta2/1 -> [DT_CAN3_SG_TM_MCUSta2]
  DT_CAN3_SG_TM_MCUSta3/1 -> [DT_CAN3_SG_TM_MCUSta3]
  [DT_CAN3_SG_B2TM_Info] -> B2TM_Info/1(DT_CAN3_SG_B2TM_Info)
  [DT_CAN3_SG_B2V_BattInfo1] -> B2V_BattInfo1/1(DT_CAN3_SG_B2V_BattInfo1)
  [DT_CAN3_SG_B2V_CurrentLimit] -> B2V_CurrentLimit/1(DT_CAN3_SG_B2V_CurrentLimit)
  [DT_CAN3_SG_B2V_Fult1_32960] -> B2V_Fult1_32960/1(DT_CAN3_SG_B2V_Fult1_32960)
  [DT_CAN3_SG_B2V_ST1] -> B2V_ST1/1(DT_CAN3_SG_B2V_ST1)
  [DT_CAN3_SG_B2V_ST2] -> B2V_ST2/1(DT_CAN3_SG_B2V_ST2)
  [DT_CAN3_SG_B2V_ST4] -> B2V_ST4/1(DT_CAN3_SG_B2V_ST4)
  [DT_CAN3_SG_B2V_ST5] -> B2V_ST5/1(DT_CAN3_SG_B2V_ST5)
  [DT_CAN3_SG_EWP1] -> EWP1/1(DT_CAN3_SG_EWP1)
  [DT_CAN3_SG_TM_MCUSta1] -> TM_MCUSta1/1(DT_CAN3_SG_TM_MCUSta1)
  [DT_CAN3_SG_TM_MCUSta2] -> TM_MCUSta2/1(DT_CAN3_SG_TM_MCUSta2)
  [DT_CAN3_SG_TM_MCUSta3] -> TM_MCUSta3/1(DT_CAN3_SG_TM_MCUSta3)
  bus_creator/1 -> HAL_CAN3_outputs/1
  VHAL_CANMsgInvalidB2TMInfo_flg/1(Out) -> bus_creator/1
  B2TM_Info/1(VHAL_B2THVRlySta_enum) -> [VHAL_B2THVRlySta_enum]
  UnitConverter/1 -> bus_creator/2  "VHAL_B2THVRlySta_enum"
  [VHAL_B2THVRlySta_enum] -> UnitConverter/1
  VHAL_CANMsgInvalidB2VBattInfo1_flg/1(Out) -> bus_creator/3
  B2V_BattInfo1/1(VHAL_B2VBI1BattType_enum) -> [VHAL_B2VBI1BattType_enum]
  UnitConverter1/1 -> bus_creator/4  "VHAL_B2VBI1BattType_enum"
  [VHAL_B2VBI1BattType_enum] -> UnitConverter1/1
  VHAL_CANMsgInvalidB2VCurrentLimit_flg/1(Out) -> bus_creator/5
  B2V_CurrentLimit/1(VHAL_B2VAPlsDischgCurr_A) -> [VHAL_B2VAPlsDischgCurr_A]
  UnitConverter2/1 -> bus_creator/6  "VHAL_B2VAPlsDischgCurr_A"
  [VHAL_B2VAPlsDischgCurr_A] -> UnitConverter2/1
  B2V_CurrentLimit/2(VHAL_B2VAvaPlsChgCurr_A) -> [VHAL_B2VAvaPlsChgCurr_A]
  UnitConverter3/1 -> bus_creator/7  "VHAL_B2VAvaPlsChgCurr_A"
  [VHAL_B2VAvaPlsChgCurr_A] -> UnitConverter3/1
  VHAL_CANMsgInvalidB2VFult132960_flg/1(Out) -> bus_creator/8
  B2V_Fult1_32960/1(VHAL_B2VHVILFault_flg) -> [VHAL_B2VHVILFault_flg]
  UnitConverter4/1 -> bus_creator/9  "VHAL_B2VHVILFault_flg"
  [VHAL_B2VHVILFault_flg] -> UnitConverter4/1
  VHAL_CANMsgInvalidB2VST1_flg/1(Out) -> bus_creator/10
  B2V_ST1/1(VHAL_B2VACChgConnSta_flg) -> [VHAL_B2VACChgConnSta_flg]
  UnitConverter5/1 -> bus_creator/11  "VHAL_B2VACChgConnSta_flg"
  [VHAL_B2VACChgConnSta_flg] -> UnitConverter5/1
  B2V_ST1/2(VHAL_B2VACChgNegRlySta_enum) -> [VHAL_B2VACChgNegRlySta_enum]
  UnitConverter6/1 -> bus_creator/12  "VHAL_B2VACChgNegRlySta_enum"
  [VHAL_B2VACChgNegRlySta_enum] -> UnitConverter6/1
  B2V_ST1/3(VHAL_B2VACChgPosRlySta_enum) -> [VHAL_B2VACChgPosRlySta_enum]
  UnitConverter7/1 -> bus_creator/13  "VHAL_B2VACChgPosRlySta_enum"
  [VHAL_B2VACChgPosRlySta_enum] -> UnitConverter7/1
  B2V_ST1/4(VHAL_B2VBMUHVSta_enum) -> [VHAL_B2VBMUHVSta_enum]
  UnitConverter8/1 -> bus_creator/14  "VHAL_B2VBMUHVSta_enum"
  [VHAL_B2VBMUHVSta_enum] -> UnitConverter8/1
  B2V_ST1/5(VHAL_B2VChgMode_enum) -> [VHAL_B2VChgMode_enum]
  UnitConverter9/1 -> bus_creator/15  "VHAL_B2VChgMode_enum"
  [VHAL_B2VChgMode_enum] -> UnitConverter9/1
  B2V_ST1/6(VHAL_B2VChgSta_enum) -> [VHAL_B2VChgSta_enum]
  UnitConverter10/1 -> bus_creator/16  "VHAL_B2VChgSta_enum"
  [VHAL_B2VChgSta_enum] -> UnitConverter10/1
  B2V_ST1/7(VHAL_B2VDCChgConnSta_enum) -> [VHAL_B2VDCChgConnSta_enum]
  UnitConverter11/1 -> bus_creator/17  "VHAL_B2VDCChgConnSta_enum"
  [VHAL_B2VDCChgConnSta_enum] -> UnitConverter11/1
  B2V_ST1/8(VHAL_B2VDCChgN1RlySta_enum) -> [VHAL_B2VDCChgN1RlySta_enum]
  UnitConverter12/1 -> bus_creator/18  "VHAL_B2VDCChgN1RlySta_enum"
  [VHAL_B2VDCChgN1RlySta_enum] -> UnitConverter12/1
  B2V_ST1/9(VHAL_B2VDCChgP1RlySta_enum) -> [VHAL_B2VDCChgP1RlySta_enum]
  UnitConverter13/1 -> bus_creator/19  "VHAL_B2VDCChgP1RlySta_enum"
  [VHAL_B2VDCChgP1RlySta_enum] -> UnitConverter13/1
  B2V_ST1/10(VHAL_B2VMainNegRlySta_enum) -> [VHAL_B2VMainNegRlySta_enum]
  UnitConverter14/1 -> bus_creator/20  "VHAL_B2VMainNegRlySta_enum"
  [VHAL_B2VMainNegRlySta_enum] -> UnitConverter14/1
  VHAL_CANMsgInvalidB2VST2_flg/1(Out) -> bus_creator/21
  B2V_ST2/1(VHAL_B2VFaultCode_enum) -> [VHAL_B2VFaultCode_enum]
  UnitConverter15/1 -> bus_creator/22  "VHAL_B2VFaultCode_enum"
  [VHAL_B2VFaultCode_enum] -> UnitConverter15/1
  B2V_ST2/2(VHAL_B2VFaultLv_enum) -> [VHAL_B2VFaultLv_enum]
  UnitConverter16/1 -> bus_creator/23  "VHAL_B2VFaultLv_enum"
  [VHAL_B2VFaultLv_enum] -> UnitConverter16/1
  B2V_ST2/3(VHAL_B2VPackCurr_A) -> [VHAL_B2VPackCurr_A]
  UnitConverter17/1 -> bus_creator/24  "VHAL_B2VPackCurr_A"
  [VHAL_B2VPackCurr_A] -> UnitConverter17/1
  B2V_ST2/4(VHAL_B2VPackInsideVol_V) -> [VHAL_B2VPackInsideVol_V]
  UnitConverter18/1 -> bus_creator/25  "VHAL_B2VPackInsideVol_V"
  [VHAL_B2VPackInsideVol_V] -> UnitConverter18/1
  B2V_ST2/5(VHAL_B2VRqHVPwrOff_enum) -> [VHAL_B2VRqHVPwrOff_enum]
  UnitConverter19/1 -> bus_creator/26  "VHAL_B2VRqHVPwrOff_enum"
  [VHAL_B2VRqHVPwrOff_enum] -> UnitConverter19/1
  B2V_ST2/6(VHAL_B2VSOC_pct) -> [VHAL_B2VSOC_pct]
  UnitConverter20/1 -> bus_creator/27  "VHAL_B2VSOC_pct"
  [VHAL_B2VSOC_pct] -> UnitConverter20/1
  VHAL_CANMsgInvalidB2VST4_flg/1(Out) -> bus_creator/28
  B2V_ST4/1(VHAL_B2VMinTempPos_enum) -> [VHAL_B2VMinTempPos_enum]
  UnitConverter21/1 -> bus_creator/29  "VHAL_B2VMinTempPos_enum"
  [VHAL_B2VMinTempPos_enum] -> UnitConverter21/1
  VHAL_CANMsgInvalidB2VST5_flg/1(Out) -> bus_creator/30
  B2V_ST5/1(VHAL_B2VCellMinVol_V) -> [VHAL_B2VCellMinVol_V]
  UnitConverter22/1 -> bus_creator/31  "VHAL_B2VCellMinVol_V"
  [VHAL_B2VCellMinVol_V] -> UnitConverter22/1
  VHAL_CANMsgInvalidEWP1_flg/1(Out) -> bus_creator/32
  EWP1/1(VHAL_EWPPEFault_enum) -> [VHAL_EWPPEFault_enum]
  UnitConverter23/1 -> bus_creator/33  "VHAL_EWPPEFault_enum"
  [VHAL_EWPPEFault_enum] -> UnitConverter23/1
  VHAL_CANMsgInvalidTMMCUSta1_flg/1(Out) -> bus_creator/34
  TM_MCUSta1/1(VHAL_AtvDisChgEnFbk_flg) -> [VHAL_AtvDisChgEnFbk_flg]
  UnitConverter24/1 -> bus_creator/35  "VHAL_AtvDisChgEnFbk_flg"
  [VHAL_AtvDisChgEnFbk_flg] -> UnitConverter24/1
  TM_MCUSta1/2(VHAL_MCUCtrlMdSta_enum) -> [VHAL_MCUCtrlMdSta_enum]
  UnitConverter25/1 -> bus_creator/36  "VHAL_MCUCtrlMdSta_enum"
  [VHAL_MCUCtrlMdSta_enum] -> UnitConverter25/1
  TM_MCUSta1/3(VHAL_MCUIGBTEnFbk_flg) -> [VHAL_MCUIGBTEnFbk_flg]
  UnitConverter26/1 -> bus_creator/37  "VHAL_MCUIGBTEnFbk_flg"
  [VHAL_MCUIGBTEnFbk_flg] -> UnitConverter26/1
  TM_MCUSta1/4(VHAL_MotorSpd_rpm) -> [VHAL_MotorSpd_rpm]
  UnitConverter27/1 -> bus_creator/38  "VHAL_MotorSpd_rpm"
  [VHAL_MotorSpd_rpm] -> UnitConverter27/1
  TM_MCUSta1/5(VHAL_MotorTrq_Nm) -> [VHAL_MotorTrq_Nm]
  UnitConverter28/1 -> bus_creator/39  "VHAL_MotorTrq_Nm"
  [VHAL_MotorTrq_Nm] -> UnitConverter28/1
  VHAL_CANMsgInvalidTMMCUSta2_flg/1(Out) -> bus_creator/40
  TM_MCUSta2/1(VHAL_MCUFailGrade_enum) -> [VHAL_MCUFailGrade_enum]
  UnitConverter29/1 -> bus_creator/41  "VHAL_MCUFailGrade_enum"
  [VHAL_MCUFailGrade_enum] -> UnitConverter29/1
  TM_MCUSta2/2(VHAL_MCUTemp_C) -> [VHAL_MCUTemp_C]
  UnitConverter30/1 -> bus_creator/42  "VHAL_MCUTemp_C"
  [VHAL_MCUTemp_C] -> UnitConverter30/1
  TM_MCUSta2/3(VHAL_MCUTrqLimHi_Nm) -> [VHAL_MCUTrqLimHi_Nm]
  UnitConverter31/1 -> bus_creator/43  "VHAL_MCUTrqLimHi_Nm"
  [VHAL_MCUTrqLimHi_Nm] -> UnitConverter31/1
  TM_MCUSta2/4(VHAL_MCUTrqLimLo_Nm) -> [VHAL_MCUTrqLimLo_Nm]
  UnitConverter32/1 -> bus_creator/44  "VHAL_MCUTrqLimLo_Nm"
  [VHAL_MCUTrqLimLo_Nm] -> UnitConverter32/1
  TM_MCUSta2/5(VHAL_MotorTemp_C) -> [VHAL_MotorTemp_C]
  UnitConverter33/1 -> bus_creator/45  "VHAL_MotorTemp_C"
  [VHAL_MotorTemp_C] -> UnitConverter33/1
  VHAL_CANMsgInvalidTMMCUSta3_flg/1(Out) -> bus_creator/46
  TM_MCUSta3/1(VHAL_MCUDCCur_A) -> [VHAL_MCUDCCur_A]
  UnitConverter34/1 -> bus_creator/47  "VHAL_MCUDCCur_A"
  [VHAL_MCUDCCur_A] -> UnitConverter34/1
  TM_MCUSta3/2(VHAL_MCUDCVol_V) -> [VHAL_MCUDCVol_V]
  UnitConverter35/1 -> bus_creator/48  "VHAL_MCUDCVol_V"
  [VHAL_MCUDCVol_V] -> UnitConverter35/1
  TM_MCUSta3/3(VHAL_MCUFailCode_enum) -> [VHAL_MCUFailCode_enum]
  UnitConverter36/1 -> bus_creator/49  "VHAL_MCUFailCode_enum"
  [VHAL_MCUFailCode_enum] -> UnitConverter36/1

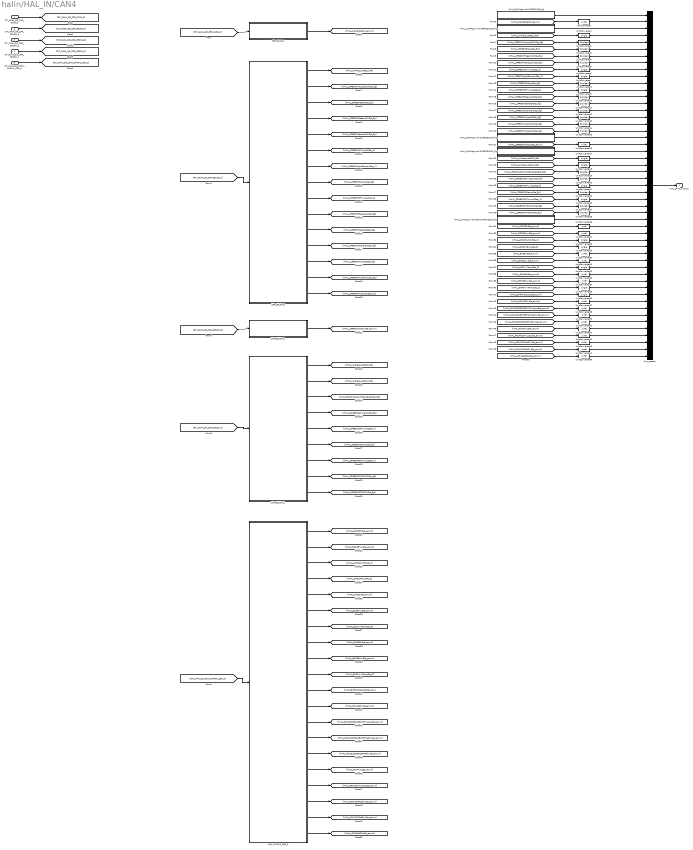
== system halin/HAL_IN/CAN4 ==
  DT_CAN4_SG_ZFR_C100_0 : Inport
  DT_CAN4_SG_ZFR_CE100_0 : Inport  Port=2
  DT_CAN4_SG_ZRR_CE100_0 : Inport  Port=3
  DT_CAN4_SG_ZRR_CE100_1 : Inport  Port=4
  DT_CAN4_SG_zGW_CANRr1_C50_0 : Inport  Port=5
  UnitConverter{,16,26..27,30..31,33..34,37..45} (17 alike) : DataTypeConversion  OutDataTypeStr=uint8
  UnitConverter{1,6..7,9,17..18,21,23,28..29,32,35..36} (13 alike) : DataTypeConversion  OutDataTypeStr=single
  UnitConverter{2..5,8,10..15,19..20,22,24..25} (16 alike) : DataTypeConversion  OutDataTypeStr=boolean
  VHAL_CANMsgInvalidZFRC1000_flg : Subsystem  AncestorBlock=FVT_lib/hal/MsgTimeoutJudge_CAN_AUTOSAR
      mask help: MeasumentTrigerEvent
      mask Display: fprintf('MsgTimeoutJudge_CAN\nAUTOSAR');
  VHAL_CANMsgInvalidZFRCE1000_flg : Subsystem  AncestorBlock=FVT_lib/hal/MsgTimeoutJudge_CAN_AUTOSAR
      mask help: MeasumentTrigerEvent
      mask Display: fprintf('MsgTimeoutJudge_CAN\nAUTOSAR');
  VHAL_CANMsgInvalidZRRCE1000_flg : Subsystem  AncestorBlock=FVT_lib/hal/MsgTimeoutJudge_CAN_AUTOSAR
      mask help: MeasumentTrigerEvent
      mask Display: fprintf('MsgTimeoutJudge_CAN\nAUTOSAR');
  VHAL_CANMsgInvalidZRRCE1001_flg : Subsystem  AncestorBlock=FVT_lib/hal/MsgTimeoutJudge_CAN_AUTOSAR
      mask help: MeasumentTrigerEvent
      mask Display: fprintf('MsgTimeoutJudge_CAN\nAUTOSAR');
  VHAL_CANMsgInvalidzGWCANRr1C500_flg : Subsystem  AncestorBlock=FVT_lib/hal/MsgTimeoutJudge_CAN_AUTOSAR
      mask help: MeasumentTrigerEvent
      mask Display: fprintf('MsgTimeoutJudge_CAN\nAUTOSAR');
  ZFR_C100_0 : Subsystem
  ZFR_CE100_0 : Subsystem
  ZRR_CE100_0 : Subsystem
  ZRR_CE100_1 : Subsystem
  bus_creator : BusCreator  Inputs=51  OutDataTypeStr=Bus: BHAL_CAN4_outputs  NonVirtualBus=on
  zGW_CANRr1_C50_0 : Subsystem
  HAL_CAN4_outputs : Outport
  wires:
  DT_CAN4_SG_ZFR_C100_0/1 -> [DT_CAN4_SG_ZFR_C100_0]
  DT_CAN4_SG_ZFR_CE100_0/1 -> [DT_CAN4_SG_ZFR_CE100_0]
  DT_CAN4_SG_ZRR_CE100_0/1 -> [DT_CAN4_SG_ZRR_CE100_0]
  DT_CAN4_SG_ZRR_CE100_1/1 -> [DT_CAN4_SG_ZRR_CE100_1]
  DT_CAN4_SG_zGW_CANRr1_C50_0/1 -> [DT_CAN4_SG_zGW_CANRr1_C50_0]
  [DT_CAN4_SG_ZFR_C100_0] -> ZFR_C100_0/1(DT_CAN4_SG_ZFR_C100_0)
  [DT_CAN4_SG_ZFR_CE100_0] -> ZFR_CE100_0/1(DT_CAN4_SG_ZFR_CE100_0)
  [DT_CAN4_SG_ZRR_CE100_0] -> ZRR_CE100_0/1(DT_CAN4_SG_ZRR_CE100_0)
  [DT_CAN4_SG_ZRR_CE100_1] -> ZRR_CE100_1/1(DT_CAN4_SG_ZRR_CE100_1)
  [DT_CAN4_SG_zGW_CANRr1_C50_0] -> zGW_CANRr1_C50_0/1(DT_CAN4_SG_zGW_CANRr1_C50_0)
  bus_creator/1 -> HAL_CAN4_outputs/1
  VHAL_CANMsgInvalidZFRC1000_flg/1(Out) -> bus_creator/1
  ZFR_C100_0/1(VHAL_ParkBrakeSW_enum) -> [VHAL_ParkBrakeSW_enum]
  UnitConverter/1 -> bus_creator/2  "VHAL_ParkBrakeSW_enum"
  [VHAL_ParkBrakeSW_enum] -> UnitConverter/1
  VHAL_CANMsgInvalidZFRCE1000_flg/1(Out) -> bus_creator/3
  ZFR_CE100_0/1(VHAL_AirPressureFC2_kPa) -> [VHAL_AirPressureFC2_kPa]
  UnitConverter1/1 -> bus_creator/4  "VHAL_AirPressureFC2_kPa"
  [VHAL_AirPressureFC2_kPa] -> UnitConverter1/1
  ZFR_CE100_0/2(VHAL_ZFRBCMAutoLightSWSta_flg) -> [VHAL_ZFRBCMAutoLightSWSta_flg]
  UnitConverter2/1 -> bus_creator/5  "VHAL_ZFRBCMAutoLightSWSta_flg"
  [VHAL_ZFRBCMAutoLightSWSta_flg] -> UnitConverter2/1
  ZFR_CE100_0/3(VHAL_ZFRBCMBrakeSta_flg) -> [VHAL_ZFRBCMBrakeSta_flg]
  UnitConverter3/1 -> bus_creator/6  "VHAL_ZFRBCMBrakeSta_flg"
  [VHAL_ZFRBCMBrakeSta_flg] -> UnitConverter3/1
  ZFR_CE100_0/4(VHAL_ZFRBCMHBeamSWSta_flg) -> [VHAL_ZFRBCMHBeamSWSta_flg]
  UnitConverter4/1 -> bus_creator/7  "VHAL_ZFRBCMHBeamSWSta_flg"
  [VHAL_ZFRBCMHBeamSWSta_flg] -> UnitConverter4/1
  ZFR_CE100_0/5(VHAL_ZFRBCMHeadLpSWSta_flg) -> [VHAL_ZFRBCMHeadLpSWSta_flg]
  UnitConverter5/1 -> bus_creator/8  "VHAL_ZFRBCMHeadLpSWSta_flg"
  [VHAL_ZFRBCMHeadLpSWSta_flg] -> UnitConverter5/1
  ZFR_CE100_0/6(VHAL_ZFRBCMLFTurnLpCSta_A) -> [VHAL_ZFRBCMLFTurnLpCSta_A]
  UnitConverter6/1 -> bus_creator/9  "VHAL_ZFRBCMLFTurnLpCSta_A"
  [VHAL_ZFRBCMLFTurnLpCSta_A] -> UnitConverter6/1
  ZFR_CE100_0/7(VHAL_ZFRBCMLightSensorVSta_V) -> [VHAL_ZFRBCMLightSensorVSta_V]
  UnitConverter7/1 -> bus_creator/10  "VHAL_ZFRBCMLightSensorVSta_V"
  [VHAL_ZFRBCMLightSensorVSta_V] -> UnitConverter7/1
  ZFR_CE100_0/8(VHAL_ZFRBCMPLampSta_flg) -> [VHAL_ZFRBCMPLampSta_flg]
  UnitConverter8/1 -> bus_creator/11  "VHAL_ZFRBCMPLampSta_flg"
  [VHAL_ZFRBCMPLampSta_flg] -> UnitConverter8/1
  ZFR_CE100_0/9(VHAL_ZFRBCMRFTurnLpCSta_A) -> [VHAL_ZFRBCMRFTurnLpCSta_A]
  UnitConverter9/1 -> bus_creator/12  "VHAL_ZFRBCMRFTurnLpCSta_A"
  [VHAL_ZFRBCMRFTurnLpCSta_A] -> UnitConverter9/1
  ZFR_CE100_0/10(VHAL_ZFRBCMRFogLpSWSta_flg) -> [VHAL_ZFRBCMRFogLpSWSta_flg]
  UnitConverter10/1 -> bus_creator/13  "VHAL_ZFRBCMRFogLpSWSta_flg"
  [VHAL_ZFRBCMRFogLpSWSta_flg] -> UnitConverter10/1
  ZFR_CE100_0/11(VHAL_ZFRBCMSeatbeltSta_flg) -> [VHAL_ZFRBCMSeatbeltSta_flg]
  UnitConverter11/1 -> bus_creator/14  "VHAL_ZFRBCMSeatbeltSta_flg"
  [VHAL_ZFRBCMSeatbeltSta_flg] -> UnitConverter11/1
  ZFR_CE100_0/12(VHAL_ZFRBCMWasherSWSta_flg) -> [VHAL_ZFRBCMWasherSWSta_flg]
  UnitConverter12/1 -> bus_creator/15  "VHAL_ZFRBCMWasherSWSta_flg"
  [VHAL_ZFRBCMWasherSWSta_flg] -> UnitConverter12/1
  ZFR_CE100_0/13(VHAL_ZFRBCMWiperASSta_flg) -> [VHAL_ZFRBCMWiperASSta_flg]
  UnitConverter13/1 -> bus_creator/16  "VHAL_ZFRBCMWiperASSta_flg"
  [VHAL_ZFRBCMWiperASSta_flg] -> UnitConverter13/1
  ZFR_CE100_0/14(VHAL_ZFRBCMWiperHSWSta_flg) -> [VHAL_ZFRBCMWiperHSWSta_flg]
  UnitConverter14/1 -> bus_creator/17  "VHAL_ZFRBCMWiperHSWSta_flg"
  [VHAL_ZFRBCMWiperHSWSta_flg] -> UnitConverter14/1
  ZFR_CE100_0/15(VHAL_ZFRBCMWiperLSWSta_flg) -> [VHAL_ZFRBCMWiperLSWSta_flg]
  UnitConverter15/1 -> bus_creator/18  "VHAL_ZFRBCMWiperLSWSta_flg"
  [VHAL_ZFRBCMWiperLSWSta_flg] -> UnitConverter15/1
  VHAL_CANMsgInvalidZRRCE1000_flg/1(Out) -> bus_creator/19
  ZRR_CE100_0/1(VHAL_ZRRBCMAllDoorSta_enum) -> [VHAL_ZRRBCMAllDoorSta_enum]
  UnitConverter16/1 -> bus_creator/20  "VHAL_ZRRBCMAllDoorSta_enum"
  [VHAL_ZRRBCMAllDoorSta_enum] -> UnitConverter16/1
  VHAL_CANMsgInvalidZRRCE1001_flg/1(Out) -> bus_creator/21
  ZRR_CE100_1/1(VHAL_AirPressurePC3_kPa) -> [VHAL_AirPressurePC3_kPa]
  UnitConverter17/1 -> bus_creator/22  "VHAL_AirPressurePC3_kPa"
  [VHAL_AirPressurePC3_kPa] -> UnitConverter17/1
  ZRR_CE100_1/2(VHAL_AirPressureRC1_kPa) -> [VHAL_AirPressureRC1_kPa]
  UnitConverter18/1 -> bus_creator/23  "VHAL_AirPressureRC1_kPa"
  [VHAL_AirPressureRC1_kPa] -> UnitConverter18/1
  ZRR_CE100_1/3(VHAL_FDCCHASSISVCUEACPressSta_flg) -> [VHAL_FDCCHASSISVCUEACPressSta_flg]
  UnitConverter19/1 -> bus_creator/24  "VHAL_FDCCHASSISVCUEACPressSta_flg"
  [VHAL_FDCCHASSISVCUEACPressSta_flg] -> UnitConverter19/1
  ZRR_CE100_1/4(VHAL_ZRRBCMCallingSWSta_flg) -> [VHAL_ZRRBCMCallingSWSta_flg]
  UnitConverter20/1 -> bus_creator/25  "VHAL_ZRRBCMCallingSWSta_flg"
  [VHAL_ZRRBCMCallingSWSta_flg] -> UnitConverter20/1
  ZRR_CE100_1/5(VHAL_ZRRBCMLRTurnLpCSta_A) -> [VHAL_ZRRBCMLRTurnLpCSta_A]
  UnitConverter21/1 -> bus_creator/26  "VHAL_ZRRBCMLRTurnLpCSta_A"
  [VHAL_ZRRBCMLRTurnLpCSta_A] -> UnitConverter21/1
  ZRR_CE100_1/6(VHAL_ZRRBCMPLampSta_flg) -> [VHAL_ZRRBCMPLampSta_flg]
  UnitConverter22/1 -> bus_creator/27  "VHAL_ZRRBCMPLampSta_flg"
  [VHAL_ZRRBCMPLampSta_flg] -> UnitConverter22/1
  ZRR_CE100_1/7(VHAL_ZRRBCMRRTurnLpCSta_A) -> [VHAL_ZRRBCMRRTurnLpCSta_A]
  UnitConverter23/1 -> bus_creator/28  "VHAL_ZRRBCMRRTurnLpCSta_A"
  [VHAL_ZRRBCMRRTurnLpCSta_A] -> UnitConverter23/1
  ZRR_CE100_1/8(VHAL_ZRRBCMSTOPSW2Sta_flg) -> [VHAL_ZRRBCMSTOPSW2Sta_flg]
  UnitConverter24/1 -> bus_creator/29  "VHAL_ZRRBCMSTOPSW2Sta_flg"
  [VHAL_ZRRBCMSTOPSW2Sta_flg] -> UnitConverter24/1
  ZRR_CE100_1/9(VHAL_ZRRBCMSTOPSWSta_flg) -> [VHAL_ZRRBCMSTOPSWSta_flg]
  UnitConverter25/1 -> bus_creator/30  "VHAL_ZRRBCMSTOPSWSta_flg"
  [VHAL_ZRRBCMSTOPSWSta_flg] -> UnitConverter25/1
  VHAL_CANMsgInvalidzGWCANRr1C500_flg/1(Out) -> bus_creator/31
  zGW_CANRr1_C50_0/1(VHAL_DCDCEnSta_enum) -> [VHAL_DCDCEnSta_enum]
  UnitConverter26/1 -> bus_creator/32  "VHAL_DCDCEnSta_enum"
  [VHAL_DCDCEnSta_enum] -> UnitConverter26/1
  zGW_CANRr1_C50_0/2(VHAL_DCDCErrLvSta_enum) -> [VHAL_DCDCErrLvSta_enum]
  UnitConverter27/1 -> bus_creator/33  "VHAL_DCDCErrLvSta_enum"
  [VHAL_DCDCErrLvSta_enum] -> UnitConverter27/1
  zGW_CANRr1_C50_0/3(VHAL_DCDCOutVolSta_V) -> [VHAL_DCDCOutVolSta_V]
  UnitConverter28/1 -> bus_creator/34  "VHAL_DCDCOutVolSta_V"
  [VHAL_DCDCOutVolSta_V] -> UnitConverter28/1
  zGW_CANRr1_C50_0/4(VHAL_DCDCTempSta_C) -> [VHAL_DCDCTempSta_C]
  UnitConverter29/1 -> bus_creator/35  "VHAL_DCDCTempSta_C"
  [VHAL_DCDCTempSta_C] -> UnitConverter29/1
  zGW_CANRr1_C50_0/5(VHAL_EACEnSta_enum) -> [VHAL_EACEnSta_enum]
  UnitConverter30/1 -> bus_creator/36  "VHAL_EACEnSta_enum"
  [VHAL_EACEnSta_enum] -> UnitConverter30/1
  zGW_CANRr1_C50_0/6(VHAL_EACErrLvSta_enum) -> [VHAL_EACErrLvSta_enum]
  UnitConverter31/1 -> bus_creator/37  "VHAL_EACErrLvSta_enum"
  [VHAL_EACErrLvSta_enum] -> UnitConverter31/1
  zGW_CANRr1_C50_0/7(VHAL_EACInvTempSta_C) -> [VHAL_EACInvTempSta_C]
  UnitConverter32/1 -> bus_creator/38  "VHAL_EACInvTempSta_C"
  [VHAL_EACInvTempSta_C] -> UnitConverter32/1
  zGW_CANRr1_C50_0/8(VHAL_EHPSEnSta_enum) -> [VHAL_EHPSEnSta_enum]
  UnitConverter33/1 -> bus_creator/39  "VHAL_EHPSEnSta_enum"
  [VHAL_EHPSEnSta_enum] -> UnitConverter33/1
  zGW_CANRr1_C50_0/9(VHAL_EHPSErrLvSta_enum) -> [VHAL_EHPSErrLvSta_enum]
  UnitConverter34/1 -> bus_creator/40  "VHAL_EHPSErrLvSta_enum"
  [VHAL_EHPSErrLvSta_enum] -> UnitConverter34/1
  zGW_CANRr1_C50_0/10(VHAL_EHPSInvTempSta_C) -> [VHAL_EHPSInvTempSta_C]
  UnitConverter35/1 -> bus_creator/41  "VHAL_EHPSInvTempSta_C"
  [VHAL_EHPSInvTempSta_C] -> UnitConverter35/1
  zGW_CANRr1_C50_0/11(VHAL_EHPSMotorSpdSta_rpm) -> [VHAL_EHPSMotorSpdSta_rpm]
  UnitConverter36/1 -> bus_creator/42  "VHAL_EHPSMotorSpdSta_rpm"
  [VHAL_EHPSMotorSpdSta_rpm] -> UnitConverter36/1
  zGW_CANRr1_C50_0/12(VHAL_PDUACRlySta_enum) -> [VHAL_PDUACRlySta_enum]
  UnitConverter37/1 -> bus_creator/43  "VHAL_PDUACRlySta_enum"
  [VHAL_PDUACRlySta_enum] -> UnitConverter37/1
  zGW_CANRr1_C50_0/13(VHAL_PDUDCDCEACEHPSHVLoopSta_enum) -> [VHAL_PDUDCDCEACEHPSHVLoopSta_enum]
  UnitConverter38/1 -> bus_creator/44  "VHAL_PDUDCDCEACEHPSHVLoopSta_enum"
  [VHAL_PDUDCDCEACEHPSHVLoopSta_enum] -> UnitConverter38/1
  zGW_CANRr1_C50_0/14(VHAL_PDUDCDCEACEHPSPreRlySta_enum) -> [VHAL_PDUDCDCEACEHPSPreRlySta_enum]
  UnitConverter39/1 -> bus_creator/45  "VHAL_PDUDCDCEACEHPSPreRlySta_enum"
  [VHAL_PDUDCDCEACEHPSPreRlySta_enum] -> UnitConverter39/1
  zGW_CANRr1_C50_0/15(VHAL_PDUDCDCEACEHPSRlySta_enum) -> [VHAL_PDUDCDCEACEHPSRlySta_enum]
  UnitConverter40/1 -> bus_creator/46  "VHAL_PDUDCDCEACEHPSRlySta_enum"
  [VHAL_PDUDCDCEACEHPSRlySta_enum] -> UnitConverter40/1
  zGW_CANRr1_C50_0/16(VHAL_PDUHVILSta_enum) -> [VHAL_PDUHVILSta_enum]
  UnitConverter41/1 -> bus_creator/47  "VHAL_PDUHVILSta_enum"
  [VHAL_PDUHVILSta_enum] -> UnitConverter41/1
  zGW_CANRr1_C50_0/17(VHAL_PDUMCUHVLoopSta_enum) -> [VHAL_PDUMCUHVLoopSta_enum]
  UnitConverter42/1 -> bus_creator/48  "VHAL_PDUMCUHVLoopSta_enum"
  [VHAL_PDUMCUHVLoopSta_enum] -> UnitConverter42/1
  zGW_CANRr1_C50_0/18(VHAL_PDUMCUPosRlySta_enum) -> [VHAL_PDUMCUPosRlySta_enum]
  UnitConverter43/1 -> bus_creator/49  "VHAL_PDUMCUPosRlySta_enum"
  [VHAL_PDUMCUPosRlySta_enum] -> UnitConverter43/1
  zGW_CANRr1_C50_0/19(VHAL_PDUMCUPreRlySta_enum) -> [VHAL_PDUMCUPreRlySta_enum]
  UnitConverter44/1 -> bus_creator/50  "VHAL_PDUMCUPreRlySta_enum"
  [VHAL_PDUMCUPreRlySta_enum] -> UnitConverter44/1
  zGW_CANRr1_C50_0/20(VHAL_PDUSelfChkSta_enum) -> [VHAL_PDUSelfChkSta_enum]
  UnitConverter45/1 -> bus_creator/51  "VHAL_PDUSelfChkSta_enum"
  [VHAL_PDUSelfChkSta_enum] -> UnitConverter45/1

== system halin/HAL_IN/CAN1/AC_BTMS_C1000_0 ==
  DT_CAN1_SG_AC_BTMS_C1000_0 : Inport
  ACAmbTemp : Subsystem
  bus_selector : BusSelector  OutputSignals=CAN1_ACAmbTemp
  VHAL_ACAmbTemp_C : Outport
  wires:
  DT_CAN1_SG_AC_BTMS_C1000_0/1 -> [DT_CAN1_SG_AC_BTMS_C1000_0]
  [DT_CAN1_SG_AC_BTMS_C1000_0] -> bus_selector/1
  bus_selector/1 -> ACAmbTemp/1(ACAmbTemp)  "<CAN1_ACAmbTemp>"
  ACAmbTemp/1(VHAL_ACAmbTemp_C) -> VHAL_ACAmbTemp_C/1

== system halin/HAL_IN/CAN1/AC_BTMS_C1000_1 ==
  DT_CAN1_SG_AC_BTMS_C1000_1 : Inport
  ACFanSpdSta : Subsystem
  bus_selector : BusSelector  OutputSignals=CAN1_ACFanSpdSta
  VHAL_ACFanSpdSta_enum : Outport
  wires:
  DT_CAN1_SG_AC_BTMS_C1000_1/1 -> [DT_CAN1_SG_AC_BTMS_C1000_1]
  [DT_CAN1_SG_AC_BTMS_C1000_1] -> bus_selector/1
  bus_selector/1 -> ACFanSpdSta/1(ACFanSpdSta)  "<CAN1_ACFanSpdSta>"
  ACFanSpdSta/1(VHAL_ACFanSpdSta_enum) -> VHAL_ACFanSpdSta_enum/1

== system halin/HAL_IN/CAN1/AC_BTMS_C1000_4 ==
  DT_CAN1_SG_AC_BTMS_C1000_4 : Inport
  TM2BFaultCode : Subsystem
  bus_selector : BusSelector  OutputSignals=CAN1_TM2BFaultCode
  VHAL_TM2BFaultCode_enum : Outport
  wires:
  DT_CAN1_SG_AC_BTMS_C1000_4/1 -> [DT_CAN1_SG_AC_BTMS_C1000_4]
  [DT_CAN1_SG_AC_BTMS_C1000_4] -> bus_selector/1
  bus_selector/1 -> TM2BFaultCode/1(TM2BFaultCode)  "<CAN1_TM2BFaultCode>"
  TM2BFaultCode/1(VHAL_TM2BFaultCode_enum) -> VHAL_TM2BFaultCode_enum/1

== system halin/HAL_IN/CAN1/AC_BTMS_C5000_0 ==
  DT_CAN1_SG_AC_BTMS_C5000_0 : Inport
  ACTempSetSta : Subsystem
  bus_selector : BusSelector  OutputSignals=CAN1_ACTempSetSta
  VHAL_ACTempSetSta_C : Outport
  wires:
  DT_CAN1_SG_AC_BTMS_C5000_0/1 -> [DT_CAN1_SG_AC_BTMS_C5000_0]
  [DT_CAN1_SG_AC_BTMS_C5000_0] -> bus_selector/1
  bus_selector/1 -> ACTempSetSta/1(ACTempSetSta)  "<CAN1_ACTempSetSta>"
  ACTempSetSta/1(VHAL_ACTempSetSta_C) -> VHAL_ACTempSetSta_C/1

== system halin/HAL_IN/CAN1/ASC1_A ==
  DT_CAN1_SG_ASC1_A : Inport
  ASC1KneelingInfo : Subsystem
  bus_selector : BusSelector  OutputSignals=CAN1_ASC1KneelingInfo
  VHAL_ASC1KneelingInfo_enum : Outport
  wires:
  DT_CAN1_SG_ASC1_A/1 -> [DT_CAN1_SG_ASC1_A]
  [DT_CAN1_SG_ASC1_A] -> bus_selector/1
  bus_selector/1 -> ASC1KneelingInfo/1(ASC1KneelingInfo)  "<CAN1_ASC1KneelingInfo>"
  ASC1KneelingInfo/1(VHAL_ASC1KneelingInfo_enum) -> VHAL_ASC1KneelingInfo_enum/1
